simulink library "GOcontroll_Moduline_Target"  (R2023b)
settings: Solver=ode45  StartTime=0.0  StopTime=10.0  RelTol=1e-3  EnableMultiTasking=on
PreLoadFcn:
  | compile_gocontroll_mex;
libraries: $bdroot x8, canmsglib x4, simulink x2
(part 4 of 4)

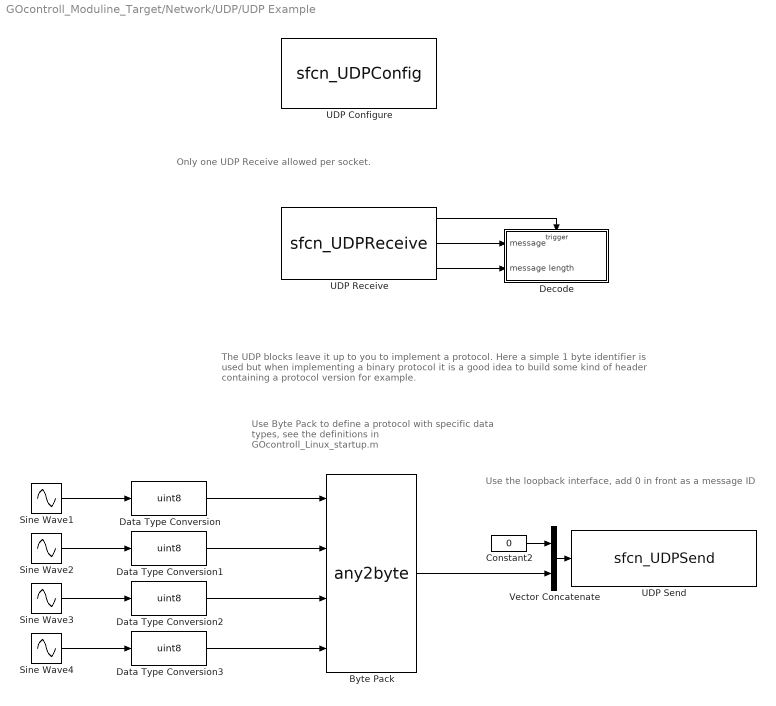
== system GOcontroll_Moduline_Target/Network/UDP/UDP Example ==
  note: The UDP blocks leave it up to you to implement a protocol.
      | Here a simple 1 byte identifier is used but when implementing a binary protocol
      | it is a good idea to build some kind of header containing a protocol version for example.
  note: Only one UDP Receive allowed per socket.
  note: Use Byte Pack to define a protocol with
      | specific data types, see the definitions in
      | GOcontroll_Linux_startup.m
  note: Use the loopback interface, add 0 in front as  a
      | message ID
  Byte Pack : S-Function  AncestorBlock=etargetslib/Byte Pack  FunctionName=any2byte  Parameters=datatypesout,byteAlign  SFunctionDeploymentMode=off  EnableBusSupport=off  mask(Byte pack){datatypes={'uint8','uint8','uint8','uint8'}, byteAlign=1}
      mask prompts: datatypes "Input port data types (cell array):"; byteAlign "Byte alignment:"
      mask help: Pack input data into a single output vector of type uint8. Insert before a UDP Send block to produce a uint8 byte vector from multiple vectors of varying data type.
      mask init:
      | datatypesout = bytepack_callback(datatypes);
      mask Help: eval('linkfoundation.util.openBlockHelp(''etargetslibbytepack'')');
      mask TypeOptions byteAlign: 1 | 2 | 4 | 8
      mask Display:
      | color('blue');
      | text(0.95, 0.90, '', ...
      |                 'horizontalalignment', 'right');
      | color('black');
      | text(0.50, 0.12, 'Byte Pack', ...
      |                 'horizontalAlignment','center');
  Constant2 : Constant  Value=0  OutDataTypeStr=uint8
  Data Type Conversion{,1..3} (4 alike) : DataTypeConversion  OutDataTypeStr=uint8  SaturateOnIntegerOverflow=off  RndMeth=Floor
  Decode : Subsystem  TreatAsAtomicUnit=on
  Sine Wave{1..4} (4 alike) : Sin  SineType=Sample based  Amplitude=120  Bias=121  Phase=128  Samples=100  SampleTime=0.01
  UDP Configure : M-S-Function  AncestorBlock=GOcontroll_Moduline_Target/Network/UDP/UDP Configure  FunctionName=sfcn_UDPConfig  mask(UDP Configure){socket_id=led_sinus, port=9001, ip='0.0.0.0', broadcast=off}
      mask prompts: socket_id "Socket id"; port "The port on which to listen/send"; ip "The ip on which to listen/send"; broadcast "Allow broadcasting of sent messages"
      mask help:
      | Block to configure a UDP connection
      |
      | Setting the ip to 0.0.0.0 makes the controller accept messages on all interfaces.
      | Set it to the ip of a specific interface to limit this.
      |
      | Allowing broadcasting enables you to send messages to a full range of ip addresses, for example:
      | 192.168.255.255 sends messages to 192.168.1.1, 192.168.2.1 ... 192.168.1.2, 192.168.1.3...
      mask init: same as GOcontroll_Moduline_Target/Network/UDP/UDP Configure
      mask Display:
      | fprintf('Configure UDP socket\n IP: %s\nPort: %d\n%s',ip,port,broadcastStr);
      | text(2, 6, ert_linux_target_version());
  UDP Receive : S-Function  AncestorBlock=GOcontroll_Moduline_Target/Network/UDP/UDP Receive  FunctionName=sfcn_UDPReceive  Parameters=buff_len,socket_id,tsamp  SFunctionDeploymentMode=off  EnableBusSupport=off  mask(UDP Receive){tsamp=-1, socket_id=led_sinus, buff_len=5}
      mask prompts: tsamp "Sample time"; socket_id "Socket"; buff_len "Buffer size"
      mask help:
      | Receive all UDP messages
      |
      | For every message received this block will call the functions attached to the function call output.
      | In these function calls you can then use the message and message length outputs to process/buffer the received messages.
      |
      | Outputs:
      | function call:
      | Attach to a function call subsystem or something like it to call that function every time a message is received.
      |
      | message:
      | The uint8 vector received from the socket. The length of this vector is likely longer than the actual number of bytes received.
      |
      | message length:
      | The number of bytes actually received, use this to get the actual fresh bytes from the message.
      |
      | Parameters:
      | buffer size:
      | The maximum number of bytes that can be read from the socket in one message, this also determines the width of the message vector.
      mask TypeOptions socket_id: id | led_sinus
      mask Callback socket_id:
      | blockPath = split(gcb, '/');
      | configures = find_system(blockPath(1),'RegExp', 'on','FollowLinks', 'on','MaskType','UDP Configure');
      | mask = Simulink.Mask.get(gcb);
      | pars = mask.Parameters;
      | options = cell(1,length(configures));
      | for idx = 1:length(configures)
      |     options(idx) = get_param(configures(idx),'socket_id');
      | end
      | mask.getParameter('socket_id').TypeOptions = options;
      mask Display:
      | fprintf('UDP Receive');
      | text(2, 6, ert_linux_target_version());
      | port_label('output', 1, 'function call');
      | port_label('output', 2, 'message');
      | port_label('output', 3, 'message length');
  UDP Send : M-S-Function  AncestorBlock=GOcontroll_Moduline_Target/Network/UDP/UDP Send  FunctionName=sfcn_UDPSend  Parameters=tsamp,ip,port  mask(UDP Send){socket_id=led_sinus, ip='127.0.0.1', port=9001, tsamp=0.01}
      mask prompts: socket_id "Socket"; ip "The IP address to send to"; port "The port to send to"; tsamp "Sample time"
      mask help:
      | Send a UDP message to the designated address.
      |
      | The Message input should be a uint8 vector, if you end up with a [1xn] or [nx1] matrix, use the reshape block to turn it into a vector.
      |
      | IP address should be a valid IP address as a string
      |
      | Port should be a within the range of a uint16
      mask init: same as GOcontroll_Moduline_Target/Network/UDP/UDP Send
      mask TypeOptions socket_id: led_sinus
      mask Callback socket_id:
      | blockPath = split(gcb, '/');
      | configures = find_system(blockPath(1),'RegExp', 'on','FollowLinks', 'on','MaskType','UDP Configure');
      | mask = Simulink.Mask.get(gcb);
      | pars = mask.Parameters;
      | options = cell(1,length(configures));
      | for idx = 1:length(configures)
      |     options(idx) = get_param(configures(idx),'socket_id');
      | end
      | pars(1).TypeOptions = options;
      mask Display:
      | fprintf('UDP Send\nIP: %s\nPort: %d',ip,port);
      | port_label('input', 1, 'message');
      | text(2, 6, ert_linux_target_version());
  Vector Concatenate : Concatenate
  wires:
  Vector Concatenate/1 -> UDP Send/1
  UDP Receive/3 -> Decode/2(message length)
  UDP Receive/2 -> Decode/1(message)
  UDP Receive/1 -> Decode/Trigger
  Sine Wave4/1 -> Data Type Conversion3/1
  Sine Wave1/1 -> Data Type Conversion/1
  Constant2/1 -> Vector Concatenate/1
  Sine Wave2/1 -> Data Type Conversion1/1
  Data Type Conversion1/1 -> Byte Pack/2
  Byte Pack/1 -> Vector Concatenate/2
  Data Type Conversion3/1 -> Byte Pack/4
  Sine Wave3/1 -> Data Type Conversion2/1
  Data Type Conversion/1 -> Byte Pack/1
  Data Type Conversion2/1 -> Byte Pack/3

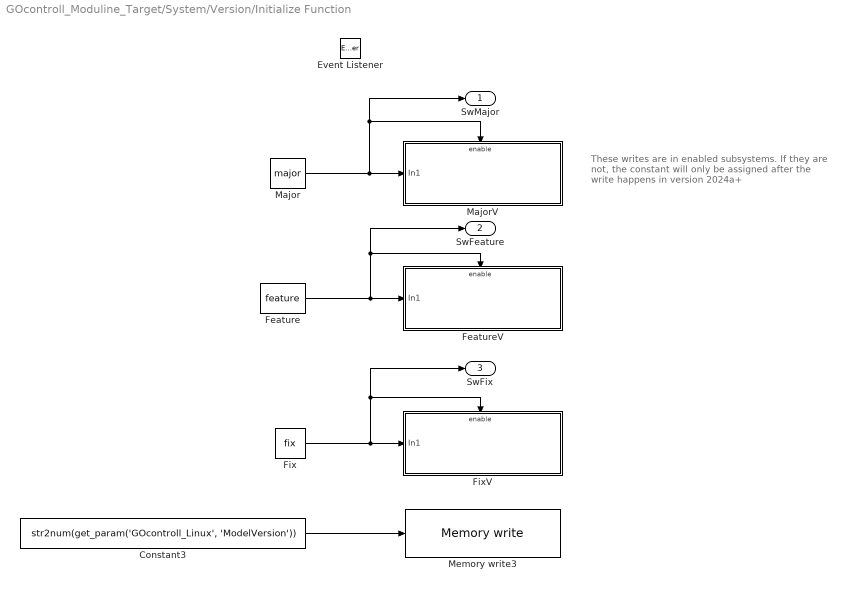
== system GOcontroll_Moduline_Target/System/Version/Initialize Function ==
  note: These writes are in enabled subsystems.
      | If they are not, the constant will only be assigned
      | after the write happens in version 2024a+
  Constant3 : Constant  Value=str2num(get_param('GOcontroll_Linux', 'ModelVersion'))  OutDataTypeStr=single
  Event Listener : EventListener  DisableCoverage=on  EventName=reset
  Feature : Constant  Value=feature  OutDataTypeStr=single
  FeatureV : Subsystem
  Fix : Constant  Value=fix  OutDataTypeStr=single
  FixV : Subsystem
  Major : Constant  Value=major  OutDataTypeStr=single
  MajorV : Subsystem
  Memory write3 : $bdroot/Memory store/Variable to memory/Memory write  memType=Persistant Memory (eMMC)  tsamp=-1  key=MODEL_BUILD
  SwMajor : Outport
  SwFeature : Outport  Port=2
  SwFix : Outport  Port=3
  wires:
  Feature/1 -> FeatureV/1(In1), SwFeature/1, FeatureV/Enable
  Constant3/1 -> Memory write3/1
  Fix/1 -> FixV/1(In1), FixV/Enable, SwFix/1
  Major/1 -> MajorV/1(In1), MajorV/Enable, SwMajor/1

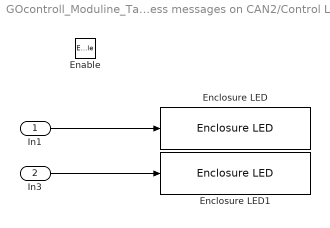
== system GOcontroll_Moduline_Target/CAN/ CAN Example/Process messages on CAN2/Control Leds ==
  In1 : Inport
  In3 : Inport  Port=2
  Enable : EnablePort
  Enclosure LED : $bdroot/Enclosure LED's/Enclosure LED  tsamp=-1  led=1  color=Blue
  Enclosure LED1 : $bdroot/Enclosure LED's/Enclosure LED  tsamp=-1  led=2  color=Blue
  wires:
  In1/1 -> Enclosure LED/1
  In3/1 -> Enclosure LED1/1

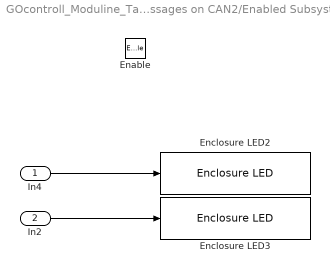
== system GOcontroll_Moduline_Target/CAN/ CAN Example/Process messages on CAN2/Enabled Subsystem ==
  In4 : Inport
  In2 : Inport  Port=2
  Enable : EnablePort
  Enclosure LED2 : $bdroot/Enclosure LED's/Enclosure LED  tsamp=-1  led=3  color=Blue
  Enclosure LED3 : $bdroot/Enclosure LED's/Enclosure LED  tsamp=-1  led=4  color=Blue
  wires:
  In4/1 -> Enclosure LED2/1
  In2/1 -> Enclosure LED3/1

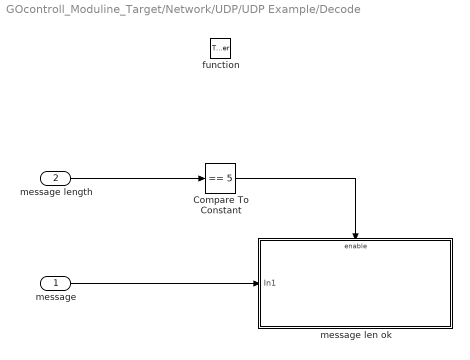
== system GOcontroll_Moduline_Target/Network/UDP/UDP Example/Decode ==
  message : Inport
  message length : Inport  Port=2
  function : TriggerPort  TriggerType=function-call  VariantControl=(inherit)
  Compare To Constant : simulink/Logic and Bit Operations/Compare To Constant  relop===  const=5  OutDataTypeStr=boolean
  message len ok : Subsystem
  wires:
  message/1 -> message len ok/1(In1)
  message length/1 -> Compare To Constant/1
  Compare To Constant/1 -> message len ok/Enable

== system GOcontroll_Moduline_Target/System/Version/Initialize Function/FeatureV ==
  In1 : Inport
  Enable : EnablePort
  Memory write1 : $bdroot/Memory store/Variable to memory/Memory write  memType=Persistant Memory (eMMC)  tsamp=-1  key=MODEL_FEATURE
  wires:
  In1/1 -> Memory write1/1

== system GOcontroll_Moduline_Target/System/Version/Initialize Function/FixV ==
  In1 : Inport
  Enable : EnablePort
  Memory write2 : $bdroot/Memory store/Variable to memory/Memory write  memType=Persistant Memory (eMMC)  tsamp=-1  key=MODEL_FIX
  wires:
  In1/1 -> Memory write2/1

== system GOcontroll_Moduline_Target/System/Version/Initialize Function/MajorV ==
  In1 : Inport
  Enable : EnablePort
  Memory write : $bdroot/Memory store/Variable to memory/Memory write  memType=Persistant Memory (eMMC)  tsamp=-1  key=MODEL_MAJOR
  wires:
  In1/1 -> Memory write/1

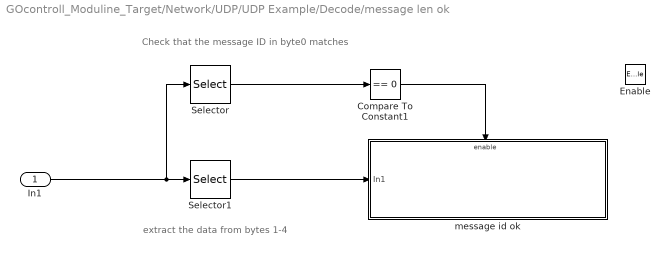
== system GOcontroll_Moduline_Target/Network/UDP/UDP Example/Decode/message len ok ==
  note: extract the data from bytes 1-4
  note: Check that the message ID in byte0 matches
  In1 : Inport
  Enable : EnablePort
  Compare To Constant1 : simulink/Logic and Bit Operations/Compare To Constant  relop===  const=0  OutDataTypeStr=boolean
  Selector : Selector  IndexMode=Zero-based  InputPortWidth=5  IndexOptions=Index vector (dialog)  Indices=[0]  OutputSizes=1
  Selector1 : Selector  IndexMode=Zero-based  InputPortWidth=5  IndexOptions=Starting index (dialog)  Indices=[1]  OutputSizes=4
  message id ok : Subsystem
  wires:
  Selector1/1 -> message id ok/1(In1)
  Selector/1 -> Compare To Constant1/1
  Compare To Constant1/1 -> message id ok/Enable
  In1/1 -> Selector/1, Selector1/1

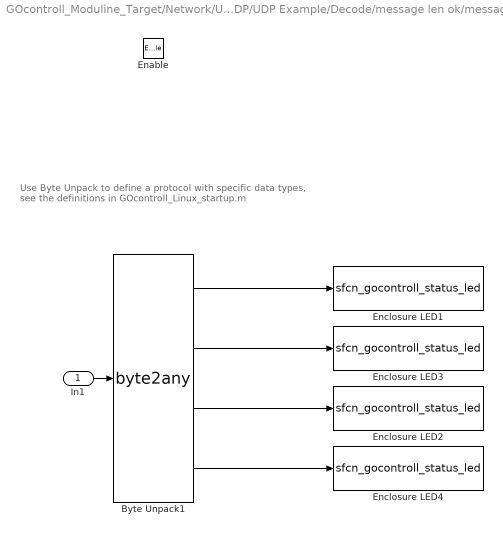
== system GOcontroll_Moduline_Target/Network/UDP/UDP Example/Decode/message len ok/message id ok ==
  note: Use Byte Unpack to define a protocol with
      | specific data types, see the definitions in
      | GOcontroll_Linux_startup.m
  In1 : Inport
  Enable : EnablePort
  Byte Unpack1 : S-Function  AncestorBlock=etargetslib/Byte Unpack  FunctionName=byte2any  Parameters=dimensionsout, datatypesout, byteAlign  SFunctionDeploymentMode=off  EnableBusSupport=off  mask(Byte Unpack){dimensions={1,1,1,1};, datatypes={'uint8','uint8','uint8','uint8'}, byteAlign=1}
      mask prompts: dimensions "Output port dimensions (cell array):"; datatypes "Output port data types (cell array):"; byteAlign "Byte alignment:"
      mask help: Unpack a binary byte vector to extract data. Insert after a UDP Recv block to break-up a UDP packet into its constituent data vectors.
      mask init:
      | [dimensionsout, datatypesout]= byteunpack_callback(dimensions, datatypes);
      mask Help: eval('linkfoundation.util.openBlockHelp(''etargetslibbyteunpack'')');
      mask TypeOptions byteAlign: 1 | 2 | 4 | 8
      mask Display:
      | color('blue');
      | text(0.95, 0.90, '', ...
      |                 'horizontalalignment', 'right');
      | color('black');
      | text(0.50, 0.12, 'Byte Unpack', ...
      |                 'horizontalAlignment','center');
  Enclosure LED1 : M-S-Function  Tag=HANcoder_TARGET_STM32_Olimexino  AncestorBlock=GOcontroll_Moduline_Target/Enclosure LED's/Enclosure LED  FunctionName=sfcn_gocontroll_status_led  Parameters=tsamp  mask(Enclosure LED's){tsamp=-1, led=1, color=Blue}
      mask prompts: tsamp "Sample time"
      mask help:
      | The Moduline controller is equipped with 4 RGB status LED's. To control them, simply configure the mask ( LED and color) and control them using uint8 values.
      |
      | Note: Moduline IV HW >= 3.02 has duty cycle controlled LED's. The intensity can be set from 0 (0%) to 255 (100%).
      |
      | LED: Select the LED that is needs to be controlled.
      |
      | Color: Select the color the LED needs to illuminate.
      mask init: same as GOcontroll_Moduline_Target/Enclosure LED's/Enclosure LED
      mask TypeOptions led: 1 | 2 | 3 | 4
      mask TypeOptions color: Red | Green | Blue
      mask Display:
      | fprintf('Status LED %d\nColor: %s',led,colorInfoStr);
      | text(2, 6, ert_linux_target_version());
  Enclosure LED2 : M-S-Function  Tag=HANcoder_TARGET_STM32_Olimexino  AncestorBlock=GOcontroll_Moduline_Target/Enclosure LED's/Enclosure LED  FunctionName=sfcn_gocontroll_status_led  Parameters=tsamp  mask(Enclosure LED's){tsamp=-1, led=3, color=Blue}
      mask prompts: tsamp "Sample time"
      mask help:
      | The Moduline controller is equipped with 4 RGB status LED's. To control them, simply configure the mask ( LED and color) and control them using uint8 values.
      |
      | Note: Moduline IV HW >= 3.02 has duty cycle controlled LED's. The intensity can be set from 0 (0%) to 255 (100%).
      |
      | LED: Select the LED that is needs to be controlled.
      |
      | Color: Select the color the LED needs to illuminate.
      mask init: same as GOcontroll_Moduline_Target/Enclosure LED's/Enclosure LED
      mask TypeOptions led: 1 | 2 | 3 | 4
      mask TypeOptions color: Red | Green | Blue
      mask Display:
      | fprintf('Status LED %d\nColor: %s',led,colorInfoStr);
      | text(2, 6, ert_linux_target_version());
  Enclosure LED3 : M-S-Function  Tag=HANcoder_TARGET_STM32_Olimexino  AncestorBlock=GOcontroll_Moduline_Target/Network/UDP/UDP Example/Decode/message len ok/message id ok/Enclosure LED2  FunctionName=sfcn_gocontroll_status_led  Parameters=tsamp  mask(Enclosure LED's){tsamp=-1, led=2, color=Blue}
      mask prompts: tsamp "Sample time"
      mask help:
      | The Moduline controller is equipped with 4 RGB status LED's. To control them, simply configure the mask ( LED and color) and control them using uint8 values.
      |
      | Note: Moduline IV HW >= 3.02 has duty cycle controlled LED's. The intensity can be set from 0 (0%) to 255 (100%).
      |
      | LED: Select the LED that is needs to be controlled.
      |
      | Color: Select the color the LED needs to illuminate.
      mask init: same as GOcontroll_Moduline_Target/Enclosure LED's/Enclosure LED
      mask TypeOptions led: 1 | 2 | 3 | 4
      mask TypeOptions color: Red | Green | Blue
      mask Display:
      | fprintf('Status LED %d\nColor: %s',led,colorInfoStr);
      | text(2, 6, ert_linux_target_version());
  Enclosure LED4 : M-S-Function  Tag=HANcoder_TARGET_STM32_Olimexino  AncestorBlock=GOcontroll_Moduline_Target/Network/UDP/UDP Example/Decode/message len ok/message id ok/Enclosure LED3  FunctionName=sfcn_gocontroll_status_led  Parameters=tsamp  mask(Enclosure LED's){tsamp=-1, led=4, color=Blue}
      mask prompts: tsamp "Sample time"
      mask help:
      | The Moduline controller is equipped with 4 RGB status LED's. To control them, simply configure the mask ( LED and color) and control them using uint8 values.
      |
      | Note: Moduline IV HW >= 3.02 has duty cycle controlled LED's. The intensity can be set from 0 (0%) to 255 (100%).
      |
      | LED: Select the LED that is needs to be controlled.
      |
      | Color: Select the color the LED needs to illuminate.
      mask init: same as GOcontroll_Moduline_Target/Enclosure LED's/Enclosure LED
      mask TypeOptions led: 1 | 2 | 3 | 4
      mask TypeOptions color: Red | Green | Blue
      mask Display:
      | fprintf('Status LED %d\nColor: %s',led,colorInfoStr);
      | text(2, 6, ert_linux_target_version());
  wires:
  In1/1 -> Byte Unpack1/1
  Byte Unpack1/2 -> Enclosure LED3/1
  Byte Unpack1/1 -> Enclosure LED1/1
  Byte Unpack1/3 -> Enclosure LED2/1
  Byte Unpack1/4 -> Enclosure LED4/1
